simulink model "ForwardIS95_Versiona"  (R2018a)
settings: Solver=FixedStepAuto  StartTime=0.0  StopTime=N*Tb  FixedStep=Tsampling  RelTol=1e-3
values from neighbouring files (symbols this model uses):
  Eb = 2    [Script_Config.m]
  fc = Rc    (= 1228800)    [Script_Config.m]
  L = K+1    (= 4)    [Script_Config.m]
  PolconSal1 = 'x^3+x'    [Script_Config.m]
  PolconSal2 = 'x^3+x^2+1'    [Script_Config.m]
  Rc = 1.2288*10^6    (= 1228800)    [Script_Config.m]
  Tb = 1/Rb    (= 0.000104166666667)    [Script_Config.m]
  Tc = 1/Rc    (= 8.13802083333e-07)    [Script_Config.m]
  Tcodif = Tb/2    (= 5.20833333333e-05)    [Script_Config.m]
  Tsampling = Tc/100    (= 8.13802083333e-09)    [Script_Config.m]
libraries: commseqgen3 x12, commdigbbndpm3 x6, commutil2 x4, commrandsrc3 x2, commcnvcod2 x2, commfilt2 x2, simulink x2
settings Model: Creator=lukit  LastModifiedBy=lukit
settings DebuggingCC: LibraryContextMissingDiagnostic=warning
settings SFSimCC: SimUseLocalCustomCode=on
settings RTWCC: RTWUseLocalCustomCode=on

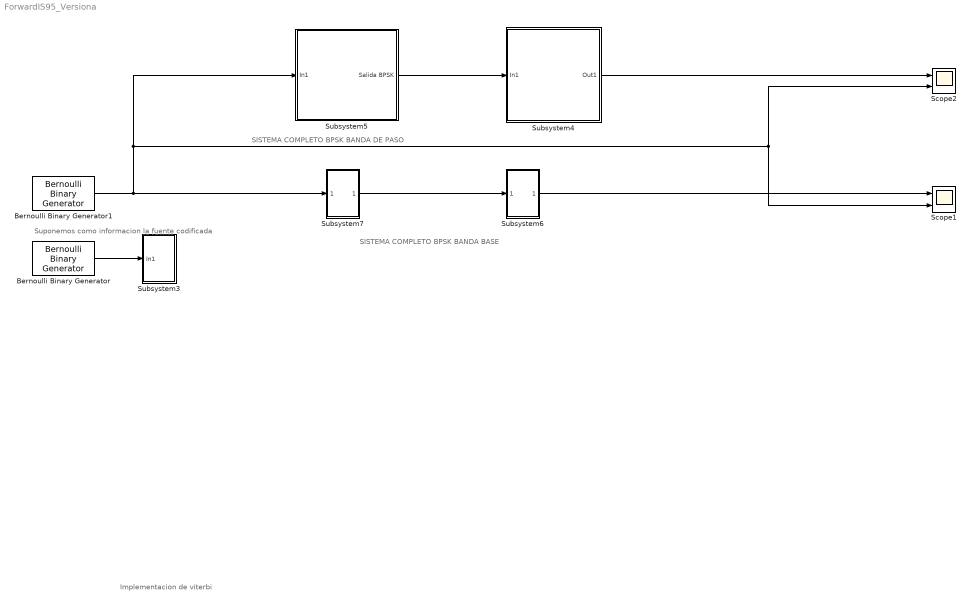
== system ForwardIS95_Versiona ==
  note: Suponemos como informacion la fuente codificada
  note: Implementacion de viterbi
  note: SISTEMA COMPLETO BPSK BANDA BASE
  note: SISTEMA COMPLETO BPSK BANDA DE PASO
  Bernoulli Binary Generator : commrandsrc3/Bernoulli Binary Generator  ProbabilityOfZero=0.5  SeedSource=Auto  Seed=0  SampleTime=Tb  SamplesPerFrame=1  OutputDataType=double  SimulateUsing=Interpreted execution
  Bernoulli Binary Generator1 : commrandsrc3/Bernoulli Binary Generator  ProbabilityOfZero=0.5  SeedSource=Auto  Seed=0  SampleTime=Tcodif  SamplesPerFrame=1  OutputDataType=double  SimulateUsing=Interpreted execution
  Scope1 : Scope  NumInputPorts=2
  Scope2 : Scope  NumInputPorts=2
  Subsystem3 : Subsystem
  Subsystem4 : Subsystem
  Subsystem5 : Subsystem
  Subsystem6 : Subsystem
  Subsystem7 : Subsystem
  wires:
  Bernoulli Binary Generator/1 -> Subsystem3/1(In1)
  Subsystem6/1(Out1) -> Scope1/1
  Subsystem7/1(Out1) -> Subsystem6/1(In1)
  Subsystem5/1(Salida BPSK) -> Subsystem4/1(In1)
  Bernoulli Binary Generator1/1 -> Scope2/2, Scope1/2, Subsystem5/1(In1), Subsystem7/1(In1)
  Subsystem4/1(Out1) -> Scope2/1

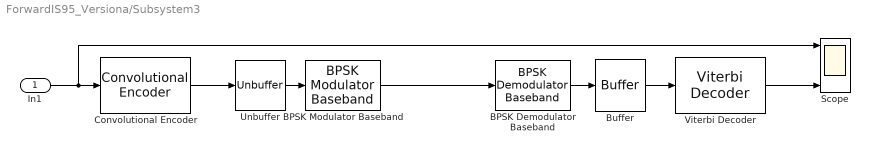
== system ForwardIS95_Versiona/Subsystem3 ==
  In1 : Inport
  BPSK Demodulator Baseband : commdigbbndpm3/BPSK Demodulator Baseband  DecType=Hard decision  VarSource=Dialog  Variance=1  Ph=0  outDtype=Inherit via internal rule  derotateFactorWordLen=16  derotateFactorDataTypeStr=Inherit: Same word length as input  derotateFactorLastDataTypeStr=Inherit: Same word length as input
  BPSK Modulator Baseband : commdigbbndpm3/BPSK Modulator Baseband  Ph=0  outDtype=double  outWordLen=16  outUDDataType=sfix(16)  outFracLenMode=Best precision  outFracLen=15  outDataTypeStr=double  outLastDataTypeStr=double
  Buffer : Buffer  N=2  OutputFrames=off
  Convolutional Encoder : commcnvcod2/Convolutional Encoder  trellis=poly2trellis(L, {PolconSal1,PolconSal2})  opMode=Continuous  DelayedResetAction=off  hasIniStPort=off  hasFinStPort=off  usePuncVector=off  punctureVector=[1; 1; 0; 1; 0; 1]  reset=Unused parameter value
      settings: SourceProductName=Communications System Toolbox  SourceProductBaseCode=CM
  Scope : Scope  NumInputPorts=3
  Unbuffer : Unbuffer
  Viterbi Decoder : commcnvcod2/Viterbi Decoder  trellis=poly2trellis(L, {PolconSal1, PolconSal2})  isPunctured=off  punctureVector=[1; 1; 0; 1; 0; 1]  erasures=off  dectype=Hard decision  nsdecb=4  runSigValErrCheck=off  tbdepth=34  opmode=Continuous  reset=off  delayedResetAction=off  smWordLength=16  outDataType=Inherit via internal rule
      settings: SourceProductName=Communications System Toolbox  SourceProductBaseCode=CM
  wires:
  Buffer/1 -> Viterbi Decoder/1
  In1/1 -> Scope/1, Convolutional Encoder/1
  Convolutional Encoder/1 -> Unbuffer/1
  Viterbi Decoder/1 -> Scope/3
  Unbuffer/1 -> BPSK Modulator Baseband/1
  BPSK Modulator Baseband/1 -> BPSK Demodulator Baseband/1
  BPSK Demodulator Baseband/1 -> Buffer/1

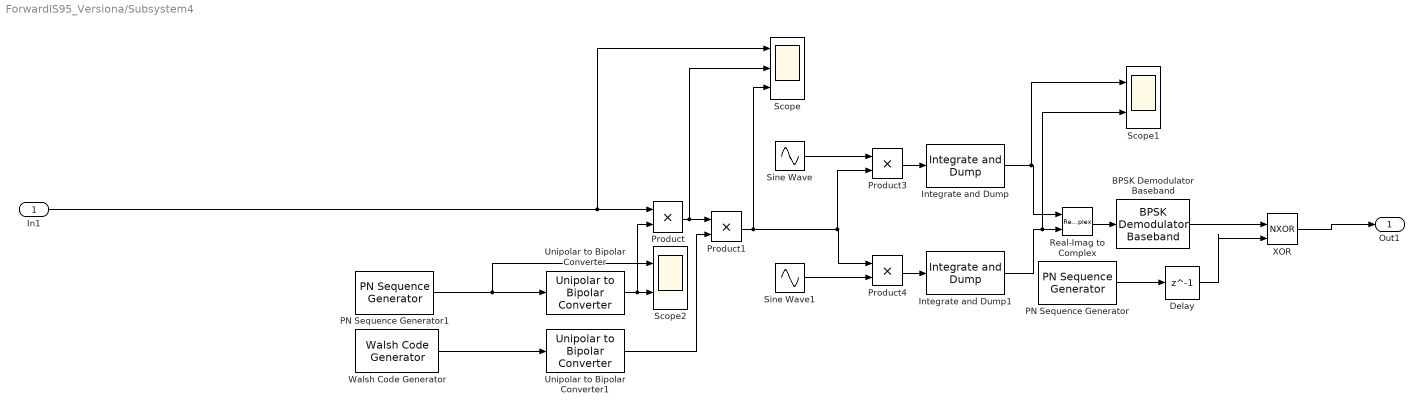
== system ForwardIS95_Versiona/Subsystem4 ==
  In1 : Inport
  BPSK Demodulator Baseband : commdigbbndpm3/BPSK Demodulator Baseband  DecType=Hard decision  VarSource=Dialog  Variance=1  Ph=0  outDtype=Inherit via internal rule  derotateFactorWordLen=16  derotateFactorDataTypeStr=Inherit: Same word length as input  derotateFactorLastDataTypeStr=Inherit: Same word length as input
  Delay : Delay  DelayLength=1  InitialCondition=0
  Integrate and Dump : commfilt2/Integrate and Dump  obssamples=TIntegracion  offsetsamples=0  nodump=off  roundingMode=Floor  overflowMode=off  outputDataTypeStr=Inherit: Same as accumulator  outputLastDataTypeStr=Inherit: Same as accumulator
      settings: SourceProductName=Communications System Toolbox
  Integrate and Dump1 : commfilt2/Integrate and Dump  obssamples=TIntegracion  offsetsamples=0  nodump=off  roundingMode=Floor  overflowMode=off  outputDataTypeStr=Inherit: Same as accumulator  outputLastDataTypeStr=Inherit: Same as accumulator
      settings: SourceProductName=Communications System Toolbox
  PN Sequence Generator : commseqgen3/PN Sequence Generator  poly=PolCodLarg  ini_sta=CondInicL  outBitMaskSource=Dialog parameter  shift=0  outVarSiz=off  maxOutSizeMode=Dialog parameter  maxOutSize=[10 1]  Ts=Tcodif  sampPerFrame=1  reset=off  bitPackedOutputs=off  outDataType=double  numPackedBits=8  bitPackDataSigned=off  bitPackedOutDType=double
      settings: SourceProductName=Communications System Toolbox
  PN Sequence Generator1 : commseqgen3/PN Sequence Generator  poly=PolCodCort  ini_sta=CondInicC  outBitMaskSource=Dialog parameter  shift=0  outVarSiz=off  maxOutSizeMode=Dialog parameter  maxOutSize=[10 1]  Ts=Tc  sampPerFrame=1  reset=off  bitPackedOutputs=off  outDataType=double  numPackedBits=8  bitPackDataSigned=off  bitPackedOutDType=double
      settings: SourceProductName=Communications System Toolbox
  Product{,1,3..4} (4 alike) : Product
  Real-Imag to Complex : RealImagToComplex
  Scope : Scope  NumInputPorts=3
  Scope1 : Scope  NumInputPorts=2
  Scope2 : Scope  NumInputPorts=2
  Sine Wave : Sin  Amplitude=sqrt(2/Tb)  Frequency=2*pi*Rc  Phase=pi/2  SampleTime=Tsampling
  Sine Wave1 : Sin  Amplitude=sqrt(2/Tb)  Frequency=2*pi*Rc  SampleTime=Tsampling
  Unipolar to Bipolar Converter : commutil2/Unipolar to Bipolar Converter  M=2  polarity=Positive  dataType=Inherit via internal rule
      settings: SourceProductName=Communications System Toolbox
  Unipolar to Bipolar Converter1 : commutil2/Unipolar to Bipolar Converter  M=2  polarity=Positive  dataType=Inherit via internal rule
      settings: SourceProductName=Communications System Toolbox
  Walsh Code Generator : commseqgen3/Walsh Code Generator  Length=64  Index=32  SampleTime=Tc  SamplesPerFrame=1  OutputDataType=double  SimulateUsing=Code generation
      settings: SourceProductName=Communications System Toolbox  SourceProductBaseCode=CM
  XOR : Logic  Operator=NXOR  IconShape=distinctive  AllPortsSameDT=off  OutDataTypeStr=boolean
  Out1 : Outport
  wires:
  PN Sequence Generator1/1 -> Scope2/1, Unipolar to Bipolar Converter/1
  Unipolar to Bipolar Converter/1 -> Scope2/2, Product/2
  Product1/1 -> Scope/3, Product3/2, Product4/1
  PN Sequence Generator/1 -> Delay/1
  Integrate and Dump1/1 -> Scope1/2, Real-Imag to Complex/2
  In1/1 -> Scope/1, Product/1
  Product3/1 -> Integrate and Dump/1
  Walsh Code Generator/1 -> Unipolar to Bipolar Converter1/1
  Product/1 -> Scope/2, Product1/1
  Real-Imag to Complex/1 -> BPSK Demodulator Baseband/1
  Unipolar to Bipolar Converter1/1 -> Product1/2
  BPSK Demodulator Baseband/1 -> XOR/1
  Sine Wave1/1 -> Product4/2
  Sine Wave/1 -> Product3/1
  Integrate and Dump/1 -> Scope1/1, Real-Imag to Complex/1
  Delay/1 -> XOR/2
  Product4/1 -> Integrate and Dump1/1
  XOR/1 -> Out1/1

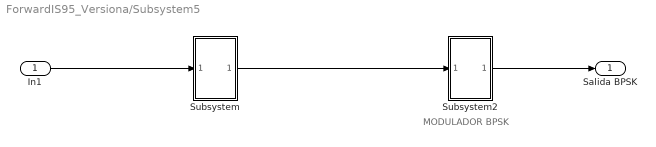
== system ForwardIS95_Versiona/Subsystem5 ==
  note: MODULADOR BPSK
  In1 : Inport
  Subsystem : Subsystem
  Subsystem2 : Subsystem
  Salida BPSK : Outport
  wires:
  In1/1 -> Subsystem/1(In1)
  Subsystem/1(Out1) -> Subsystem2/1(In1)
  Subsystem2/1(Out1) -> Salida BPSK/1

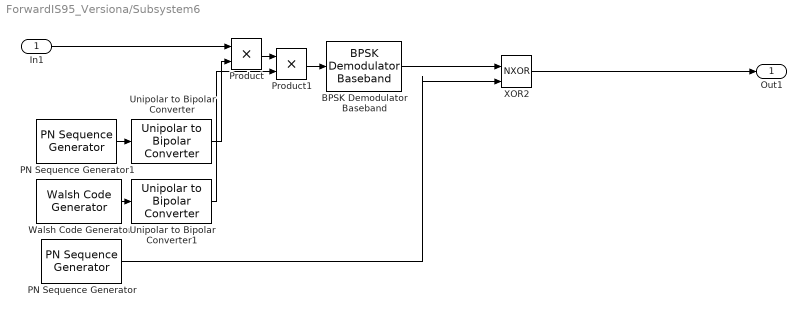
== system ForwardIS95_Versiona/Subsystem6 ==
  In1 : Inport
  BPSK Demodulator Baseband : commdigbbndpm3/BPSK Demodulator Baseband  DecType=Hard decision  VarSource=Dialog  Variance=1  Ph=0  outDtype=Inherit via internal rule  derotateFactorWordLen=16  derotateFactorDataTypeStr=Inherit: Same word length as input  derotateFactorLastDataTypeStr=Inherit: Same word length as input
  PN Sequence Generator : commseqgen3/PN Sequence Generator  poly=PolCodLarg  ini_sta=CondInicL  outBitMaskSource=Dialog parameter  shift=0  outVarSiz=off  maxOutSizeMode=Dialog parameter  maxOutSize=[10 1]  Ts=Tcodif  sampPerFrame=1  reset=off  bitPackedOutputs=off  outDataType=double  numPackedBits=8  bitPackDataSigned=off  bitPackedOutDType=double
      settings: SourceProductName=Communications System Toolbox
  PN Sequence Generator1 : commseqgen3/PN Sequence Generator  poly=PolCodCort  ini_sta=CondInicC  outBitMaskSource=Dialog parameter  shift=0  outVarSiz=off  maxOutSizeMode=Dialog parameter  maxOutSize=[10 1]  Ts=Tc  sampPerFrame=1  reset=off  bitPackedOutputs=off  outDataType=double  numPackedBits=8  bitPackDataSigned=off  bitPackedOutDType=double
      settings: SourceProductName=Communications System Toolbox
  Product : Product
  Product1 : Product
  Unipolar to Bipolar Converter : commutil2/Unipolar to Bipolar Converter  M=2  polarity=Positive  dataType=Inherit via internal rule
      settings: SourceProductName=Communications System Toolbox
  Unipolar to Bipolar Converter1 : commutil2/Unipolar to Bipolar Converter  M=2  polarity=Positive  dataType=Inherit via internal rule
      settings: SourceProductName=Communications System Toolbox
  Walsh Code Generator : commseqgen3/Walsh Code Generator  Length=64  Index=32  SampleTime=Tc  SamplesPerFrame=1  OutputDataType=double  SimulateUsing=Code generation
      settings: SourceProductName=Communications System Toolbox  SourceProductBaseCode=CM
  XOR2 : Logic  Operator=NXOR  IconShape=distinctive  AllPortsSameDT=off  OutDataTypeStr=boolean
  Out1 : Outport
  wires:
  Unipolar to Bipolar Converter/1 -> Product/2
  PN Sequence Generator/1 -> XOR2/2
  XOR2/1 -> Out1/1
  PN Sequence Generator1/1 -> Unipolar to Bipolar Converter/1
  BPSK Demodulator Baseband/1 -> XOR2/1
  Unipolar to Bipolar Converter1/1 -> Product1/2
  Product/1 -> Product1/1
  Walsh Code Generator/1 -> Unipolar to Bipolar Converter1/1
  Product1/1 -> BPSK Demodulator Baseband/1
  In1/1 -> Product/1

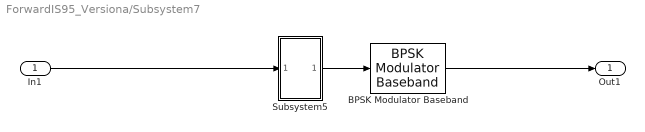
== system ForwardIS95_Versiona/Subsystem7 ==
  In1 : Inport
  BPSK Modulator Baseband : commdigbbndpm3/BPSK Modulator Baseband  Ph=0  outDtype=double  outWordLen=16  outUDDataType=sfix(16)  outFracLenMode=Best precision  outFracLen=15  outDataTypeStr=double  outLastDataTypeStr=double
  Subsystem5 : Subsystem
  Out1 : Outport
  wires:
  In1/1 -> Subsystem5/1(In1)
  Subsystem5/1(Out1) -> BPSK Modulator Baseband/1
  BPSK Modulator Baseband/1 -> Out1/1

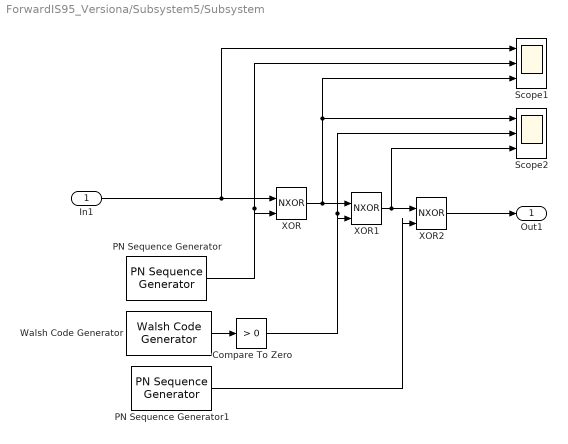
== system ForwardIS95_Versiona/Subsystem5/Subsystem ==
  In1 : Inport
  Compare To Zero : simulink/Logic and Bit Operations/Compare To Zero  relop=>  OutDataTypeStr=boolean
  PN Sequence Generator : commseqgen3/PN Sequence Generator  poly=PolCodLarg  ini_sta=CondInicL  outBitMaskSource=Dialog parameter  shift=0  outVarSiz=off  maxOutSizeMode=Dialog parameter  maxOutSize=[10 1]  Ts=Tcodif  sampPerFrame=1  reset=off  bitPackedOutputs=off  outDataType=double  numPackedBits=8  bitPackDataSigned=off  bitPackedOutDType=double
      settings: SourceProductName=Communications System Toolbox
  PN Sequence Generator1 : commseqgen3/PN Sequence Generator  poly=PolCodCort  ini_sta=CondInicC  outBitMaskSource=Dialog parameter  shift=0  outVarSiz=off  maxOutSizeMode=Dialog parameter  maxOutSize=[10 1]  Ts=Tc  sampPerFrame=1  reset=off  bitPackedOutputs=off  outDataType=double  numPackedBits=8  bitPackDataSigned=off  bitPackedOutDType=double
      settings: SourceProductName=Communications System Toolbox
  Scope1 : Scope  NumInputPorts=3
  Scope2 : Scope  NumInputPorts=3
  Walsh Code Generator : commseqgen3/Walsh Code Generator  Length=64  Index=32  SampleTime=Tc  SamplesPerFrame=1  OutputDataType=double  SimulateUsing=Code generation
      settings: SourceProductName=Communications System Toolbox  SourceProductBaseCode=CM
  XOR : Logic  Operator=NXOR  IconShape=distinctive  AllPortsSameDT=off  OutDataTypeStr=boolean
  XOR1 : Logic  Operator=NXOR  IconShape=distinctive  AllPortsSameDT=off  OutDataTypeStr=boolean
  XOR2 : Logic  Operator=NXOR  IconShape=distinctive  AllPortsSameDT=off  OutDataTypeStr=boolean
  Out1 : Outport
  wires:
  PN Sequence Generator/1 -> Scope1/2, XOR/2
  XOR1/1 -> XOR2/1, Scope2/3
  Compare To Zero/1 -> Scope2/2, XOR1/2
  In1/1 -> Scope1/1, XOR/1
  Walsh Code Generator/1 -> Compare To Zero/1
  XOR/1 -> XOR1/1, Scope2/1, Scope1/3
  XOR2/1 -> Out1/1
  PN Sequence Generator1/1 -> XOR2/2

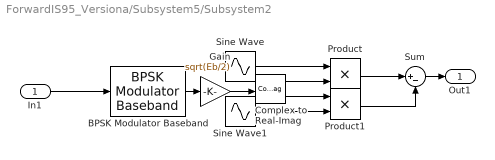
== system ForwardIS95_Versiona/Subsystem5/Subsystem2 ==
  In1 : Inport
  BPSK Modulator Baseband : commdigbbndpm3/BPSK Modulator Baseband  Ph=0  outDtype=double  outWordLen=16  outUDDataType=sfix(16)  outFracLenMode=Best precision  outFracLen=15  outDataTypeStr=double  outLastDataTypeStr=double
  Complex to Real-Imag : ComplexToRealImag
  Gain : Gain  Gain=sqrt(Eb/2)
  Product : Product
  Product1 : Product
  Sine Wave : Sin  Amplitude=sqrt(2/Tb)  Frequency=2*pi*Rc  Phase=pi/2  SampleTime=Tsampling
  Sine Wave1 : Sin  Amplitude=sqrt(2/Tb)  Frequency=2*pi*fc  SampleTime=Tsampling
  Sum : Sum  Inputs=|+-
  Out1 : Outport
  wires:
  BPSK Modulator Baseband/1 -> Gain/1
  Product/1 -> Sum/1
  Product1/1 -> Sum/2
  Gain/1 -> Complex to Real-Imag/1
  Complex to Real-Imag/1 -> Product/2
  Sine Wave/1 -> Product/1
  Sine Wave1/1 -> Product1/2
  In1/1 -> BPSK Modulator Baseband/1
  Complex to Real-Imag/2 -> Product1/1
  Sum/1 -> Out1/1

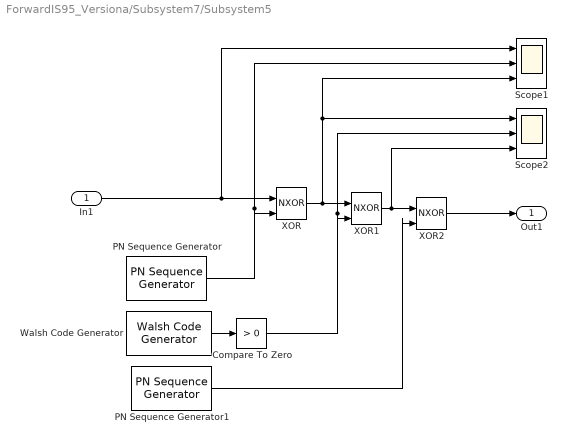
== system ForwardIS95_Versiona/Subsystem7/Subsystem5 ==
  In1 : Inport
  Compare To Zero : simulink/Logic and Bit Operations/Compare To Zero  relop=>  OutDataTypeStr=boolean
  PN Sequence Generator : commseqgen3/PN Sequence Generator  poly=PolCodLarg  ini_sta=CondInicL  outBitMaskSource=Dialog parameter  shift=0  outVarSiz=off  maxOutSizeMode=Dialog parameter  maxOutSize=[10 1]  Ts=Tcodif  sampPerFrame=1  reset=off  bitPackedOutputs=off  outDataType=double  numPackedBits=8  bitPackDataSigned=off  bitPackedOutDType=double
      settings: SourceProductName=Communications System Toolbox
  PN Sequence Generator1 : commseqgen3/PN Sequence Generator  poly=PolCodCort  ini_sta=CondInicC  outBitMaskSource=Dialog parameter  shift=0  outVarSiz=off  maxOutSizeMode=Dialog parameter  maxOutSize=[10 1]  Ts=Tc  sampPerFrame=1  reset=off  bitPackedOutputs=off  outDataType=double  numPackedBits=8  bitPackDataSigned=off  bitPackedOutDType=double
      settings: SourceProductName=Communications System Toolbox
  Scope1 : Scope  NumInputPorts=3
  Scope2 : Scope  NumInputPorts=3
  Walsh Code Generator : commseqgen3/Walsh Code Generator  Length=64  Index=32  SampleTime=Tc  SamplesPerFrame=1  OutputDataType=double  SimulateUsing=Code generation
      settings: SourceProductName=Communications System Toolbox  SourceProductBaseCode=CM
  XOR : Logic  Operator=NXOR  IconShape=distinctive  AllPortsSameDT=off  OutDataTypeStr=boolean
  XOR1 : Logic  Operator=NXOR  IconShape=distinctive  AllPortsSameDT=off  OutDataTypeStr=boolean
  XOR2 : Logic  Operator=NXOR  IconShape=distinctive  AllPortsSameDT=off  OutDataTypeStr=boolean
  Out1 : Outport
  wires:
  PN Sequence Generator/1 -> Scope1/2, XOR/2
  XOR1/1 -> XOR2/1, Scope2/3
  Compare To Zero/1 -> Scope2/2, XOR1/2
  In1/1 -> Scope1/1, XOR/1
  Walsh Code Generator/1 -> Compare To Zero/1
  XOR/1 -> XOR1/1, Scope2/1, Scope1/3
  XOR2/1 -> Out1/1
  PN Sequence Generator1/1 -> XOR2/2
